simulink model "MODEL_TESTS"  (R2024a)
settings: Solver=VariableStepAuto  StartTime=0.0  StopTime=10.0  RelTol=1e-3
values from neighbouring files (symbols this model uses):
  HEADING_AIMED_RADIANS = [0.9239;0.9202;0.6775;1.9677;2.1390;1.9622;2.8397;2.4664;2.1408;2.2191;1.8417]    [GNSS_COMPASS_LINEAR_MODEL_FUSION.m]
  INPUTS_CONTROL_B = -1    [GNSS_COMPASS_LINEAR_MODEL_FUSION.m]
  PROCESS_NOISE_CONTROL_MATRIX = INPUTS_CONTROL_B    (= -1)    [GNSS_COMPASS_LINEAR_MODEL_FUSION.m]
  STATE_MATRIX_MODEL_A = 1    [GNSS_COMPASS_LINEAR_MODEL_FUSION.m]
undefined symbols (not defined in the file or in its folder): DiscIntNeverNeededParam, PROCESS_NOISE
settings Model: Creator=gerar  LastModifiedBy=gerar

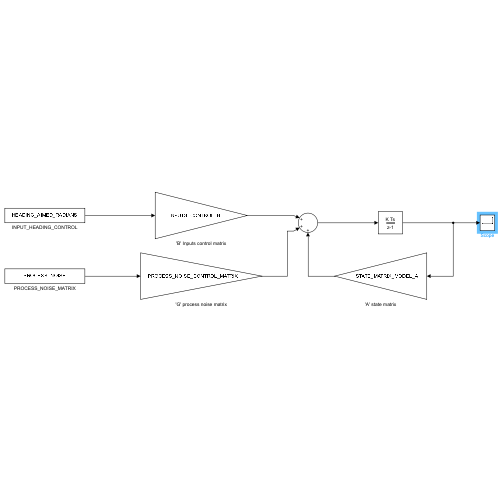
[thumbnail: Simulink's stored preview of the top-level diagram]
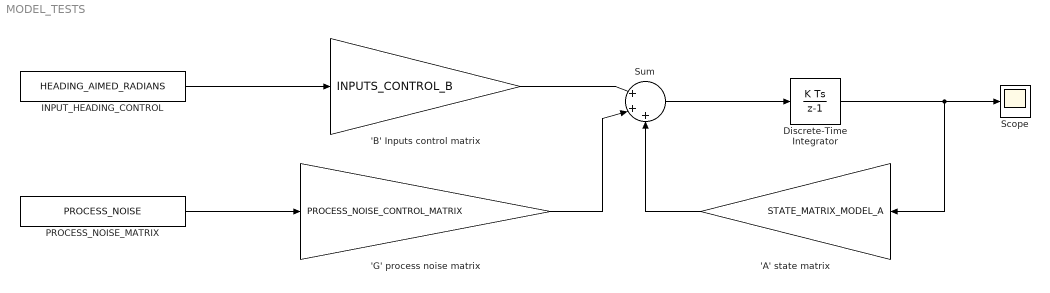
== system MODEL_TESTS ==
  'A' state matrix : Gain  Gain=STATE_MATRIX_MODEL_A
  'B' Inputs control matrix : Gain  Gain=INPUTS_CONTROL_B
  'G' process noise matrix : Gain  Gain=PROCESS_NOISE_CONTROL_MATRIX
  Discrete-Time Integrator : DiscreteIntegrator  InitialCondition=HEADING_AIMED_RADIANS(1)  SampleTime=-1  ICPrevOutput=DiscIntNeverNeededParam  ICPrevScaledInput=DiscIntNeverNeededParam
  INPUT_HEADING_CONTROL : Constant  Value=HEADING_AIMED_RADIANS
  PROCESS_NOISE_MATRIX : Constant  Value=PROCESS_NOISE
  Scope : Scope
  Sum : Sum  Inputs=|+++
  wires:
  'A' state matrix/1 -> Sum/3
  PROCESS_NOISE_MATRIX/1 -> 'G' process noise matrix/1
  'G' process noise matrix/1 -> Sum/2
  Discrete-Time Integrator/1 -> Scope/1, 'A' state matrix/1
  Sum/1 -> Discrete-Time Integrator/1
  'B' Inputs control matrix/1 -> Sum/1
  INPUT_HEADING_CONTROL/1 -> 'B' Inputs control matrix/1
